simulink model "podc"  (R2015a)
settings: Solver=ode45  StartTime=0.0  StopTime=5  RelTol=1e-3
libraries: fuzblock x1
settings Model: Creator=Sandra Knezevic  LastModifiedBy=Sandra Knezevic

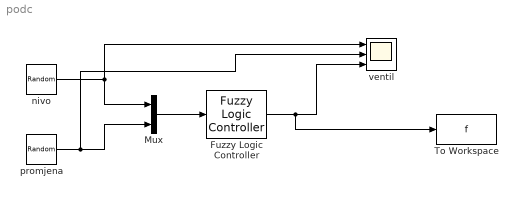
== system podc ==
  Fuzzy Logic Controller : fuzblock/Fuzzy Logic  Controller  fis=fazzi
  Mux : Mux  Inputs=2
  To Workspace : ToWorkspace  VariableName=f  SampleTime=-1
  nivo : RandomNumber  Mean=-1  SampleTime=0.1
  promjena : RandomNumber  Mean=-0.55  Variance=0.55  SampleTime=0.1
  ventil : Scope  NumInputPorts=3
      settings: TickLabels=on  ShowLegends=on  YMin=-5~-5~-5  YMax=5~5~5
  wires:
  Fuzzy Logic Controller/1 -> To Workspace/1, ventil/3
  Mux/1 -> Fuzzy Logic Controller/1
  promjena/1 -> ventil/2, Mux/2
  nivo/1 -> Mux/1, ventil/1
